simulink model "zbiornik_sys"  (R2021b)
settings: Solver=VariableStepAuto  StartTime=0.0  StopTime=10.0  RelTol=1e-3
settings Model: Creator=szczy  LastModifiedBy=szczy

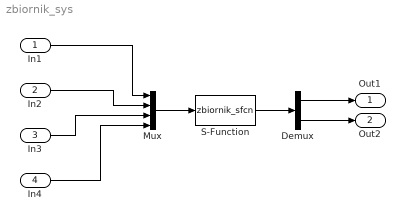
== system zbiornik_sys ==
  In1 : Inport
  In2 : Inport  Port=2
  In3 : Inport  Port=3
  In4 : Inport  Port=4
  Demux : Demux  Outputs=2
  Mux : Mux
  S-Function : S-Function  FunctionName=zbiornik_sfcn  Parameters=V0 T0  SFunctionDeploymentMode=off  EnableBusSupport=off
  Out1 : Outport
  Out2 : Outport  Port=2
  wires:
  In4/1 -> Mux/4
  In3/1 -> Mux/3
  In2/1 -> Mux/2
  In1/1 -> Mux/1
  Demux/1 -> Out1/1
  Demux/2 -> Out2/1
  Mux/1 -> S-Function/1
  S-Function/1 -> Demux/1
